simulink model "passive_Suspension"  (R2025b)
settings: Solver=VariableStepAuto  StartTime=0.0  StopTime=2.5  RelTol=1e-3
values from neighbouring files (symbols this model uses):
  c_s = 2100    [Report_Script_Suspension.m]
  k_s = 28500    [Report_Script_Suspension.m]
  k_u = 200000    [Report_Script_Suspension.m]
  m_s = (m_veh*wbf*wbl) - m_u    (= 565.5)    [Report_Script_Suspension.m]
  m_uf = 45    [Report_Script_Suspension.m]
  mph_to_ms = 0.44704    [Report_Script_Suspension.m]
  v_mph = 20    [Report_Script_Suspension.m]
undefined symbols (not defined in the file or in its folder): road_profile_change, road_surface_length
settings Model: Creator=jens.lahr  LastModifiedBy=M Wasib
settings ModelReferenceCC: EnableRefExpFcnMdlSchedulingChecks=on
settings RTWCC: GPUComputeCapability=3.5

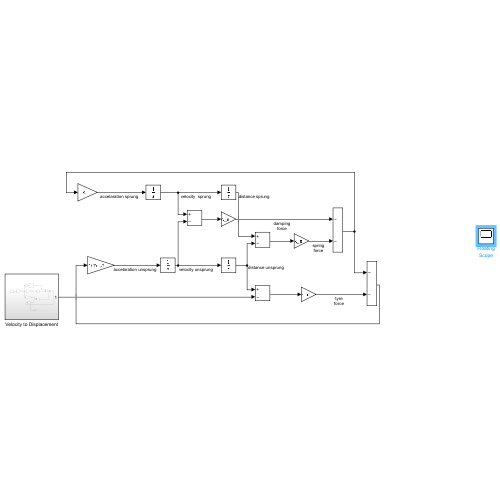
[thumbnail: Simulink's stored preview of the top-level diagram]
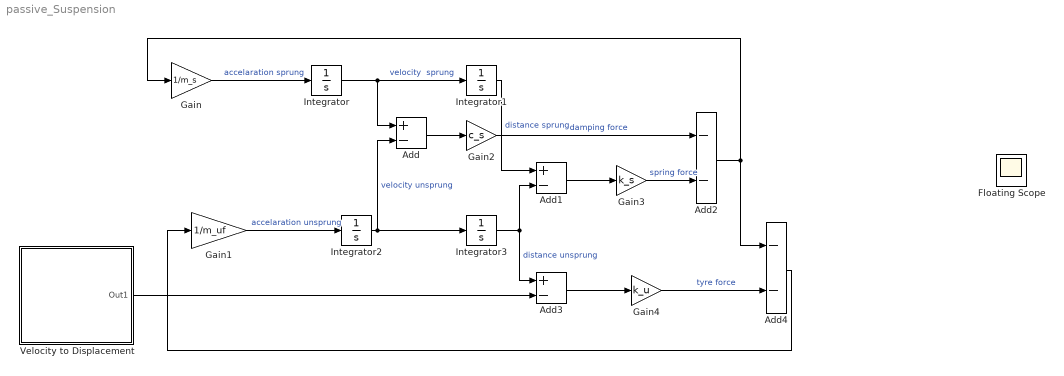
== system passive_Suspension ==
  Add : Sum  Inputs=+-
  Add1 : Sum  Inputs=+-
  Add2 : Sum  Inputs=--
  Add3 : Sum  Inputs=+-
  Add4 : Sum  Inputs=--
  Floating Scope : Scope
      settings: IsFloating=on  Floating=on  ActiveDisplayYMinimum=-0.000926727999270554  ActiveDisplayYMaximum=0.0025691790897764983
  Gain : Gain  Gain=1/m_s
  Gain1 : Gain  Gain=1/m_uf
  Gain2 : Gain  Gain=c_s
  Gain3 : Gain  Gain=k_s
  Gain4 : Gain  Gain=k_u
  Integrator{,1..3} (4 alike) : Integrator
  Velocity to Displacement : Subsystem
  wires:
  Gain/1 -> Integrator/1  "accelaration sprung"
  Integrator/1 -> Add/1, Integrator1/1  "velocity  sprung"
  Integrator1/1 -> Add1/1  "distance sprung"
  Integrator2/1 -> Add/2, Integrator3/1  "velocity unsprung"
  Gain1/1 -> Integrator2/1  "accelaration unsprung"
  Integrator3/1 -> Add3/1, Add1/2  "distance unsprung"
  Add/1 -> Gain2/1
  Add1/1 -> Gain3/1
  Gain3/1 -> Add2/2  "spring force"
  Gain2/1 -> Add2/1  "damping force"
  Add2/1 -> Add4/1, Gain/1
  Add3/1 -> Gain4/1
  Gain4/1 -> Add4/2  "tyre force"
  Add4/1 -> Gain1/1
  Velocity to Displacement/1(Out1) -> Add3/2

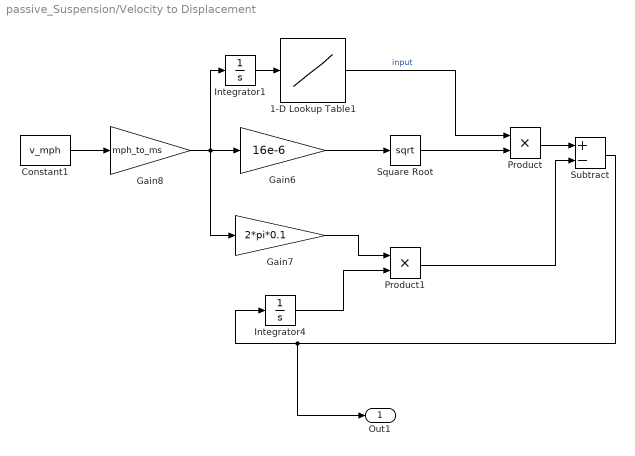
== system passive_Suspension/Velocity to Displacement ==
  1-D Lookup Table1 : Lookup_n-D  NumberOfTableDimensions=1  BreakpointsForDimension1=road_surface_length  Table=road_profile_change  InternalRulePriority=Speed  RndMeth=Simplest
  Constant1 : Constant  Value=v_mph
  Gain6 : Gain  Gain=16e-6
  Gain7 : Gain  Gain=2*pi*0.1
  Gain8 : Gain  Gain=mph_to_ms
  Integrator1 : Integrator
  Integrator4 : Integrator
  Product : Product
  Product1 : Product
  Square Root : Sqrt
  Subtract : Sum  Inputs=+-
  Out1 : Outport
  wires:
  Product/1 -> Subtract/1
  Integrator4/1 -> Product1/2
  Subtract/1 -> Out1/1, Integrator4/1
  Constant1/1 -> Gain8/1
  Product1/1 -> Subtract/2
  Square Root/1 -> Product/2
  Gain6/1 -> Square Root/1
  Gain8/1 -> Gain6/1, Gain7/1, Integrator1/1
  Integrator1/1 -> 1-D Lookup Table1/1
  1-D Lookup Table1/1 -> Product/1  "input"
  Gain7/1 -> Product1/1
